simulink model "MISSILE_SIM_ADRC"  (R2025b)
settings: Solver=VariableStepAuto  StartTime=0.0  StopTime=10.0  RelTol=1e-3
settings Model: Creator=91872  LastModifiedBy=91872

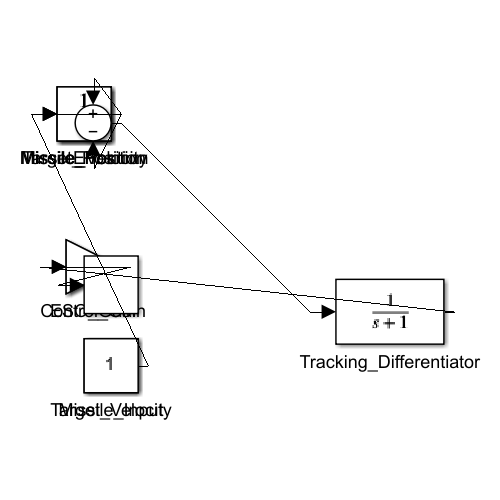
[thumbnail: Simulink's stored preview of the top-level diagram]
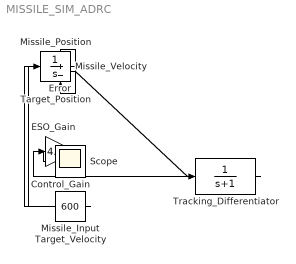
== system MISSILE_SIM_ADRC ==
  Control_Gain : Gain  Gain=14.3
  ESO_Gain : Gain  Gain=4.5
  Error : Sum  Inputs=+-
  Missile_Input : Constant
  Missile_Position : Integrator
  Missile_Velocity : Integrator
  Scope : Scope
  Target_Position : Integrator
  Target_Velocity : Constant  Value=600
  Tracking_Differentiator : TransferFcn  Denominator=[1 1]
  wires:
  Target_Velocity/1 -> Target_Position/1
  Missile_Input/1 -> Missile_Velocity/1
  Missile_Velocity/1 -> Missile_Position/1
  Target_Position/1 -> Error/1
  Missile_Position/1 -> Error/2
  Error/1 -> Tracking_Differentiator/1
  Tracking_Differentiator/1 -> ESO_Gain/1
  ESO_Gain/1 -> Control_Gain/1
  Control_Gain/1 -> Scope/1
